simulink model "model"  (R2025b)
settings: Solver=ode4  StartTime=0.0  StopTime=20  FixedStep=1e-3  RelTol=1e-3
values from neighbouring files (symbols this model uses):
  center_circ = [0,0]    [trajectories.m]
  ellipse_center = [0, 0]    [trajectories.m]
  ellipse_x_axis = 3    [trajectories.m]
  ellipse_y_axis = 1    [trajectories.m]
  K_posture = [100;100;0.01]    [posture_controllers.m]    (also in sim_FT.m = [10,10,100]; simulate_full_task.m = [10,10,100])
  KL_params = [1, 1]    [simulate_configuration_control.m]    (also in simulate_trajectory_tracking.m; tracking_controllers.m = [KL_a, KL_xi])
  KNL_b = 100    [sim_FT.m]    (also in simulate_configuration_control.m = 1; simulate_full_task.m; simulate_trajectory_tracking.m = 1; tracking_controllers.m = 1000)
  KNL_xi = 0.25    [sim_FT.m]    (also in simulate_configuration_control.m = 0.5; simulate_full_task.m; simulate_trajectory_tracking.m = 0.5; tracking_controllers.m = 0.9999)
  omega_circ = 1    [trajectories.m]
  q0_posture = [err_mag;err_phase;delta_pos]    [posture_controllers.m]    (also in sim_FT.m = [rho_0; gamma_0; delta_0]; simulate_configuration_control.m; simulate_full_task.m = [rho_0; gamma_0; delta_0])
  q_h_0 = [x_h_0, y_h, theta_h]    [trajectories.m]
  q_h_f = [x_h_f, y_h, theta_h]    [trajectories.m]
  q_v_0 = [x_v, y_v_0, theta_v]    [trajectories.m]
  q_v_f = [x_v, y_v_f, theta_v]    [trajectories.m]
  R_circ = 1    [trajectories.m]
  x0_cartesian = [-1;-1;pi/4]    [posture_controllers.m]    (also in simulate_configuration_control.m)
  zigzag_ampl = 3    [trajectories.m]
  zigzag_period = 6    [trajectories.m]
  zigzag_period_length = 3    [trajectories.m]
settings Model: Creator=llp  LastModifiedBy=fede

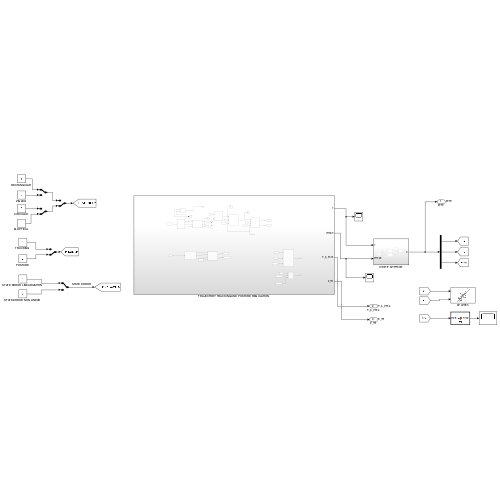
[thumbnail: Simulink's stored preview of the top-level diagram]
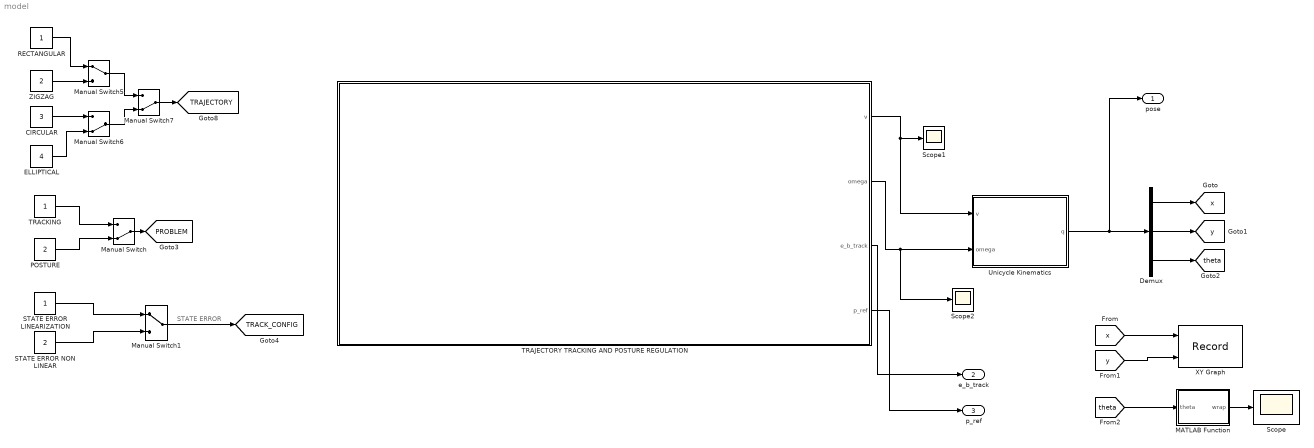
== system model ==
  note: STATE ERROR
  CIRCULAR : Constant  Value=3
  Demux : Demux  Outputs=3
  ELLIPTICAL : Constant  Value=4
  MATLAB Function : MATLAB Function  TreatAsAtomicUnit=on
  Manual Switch : ManualSwitch  CurrentSetting=0
  Manual Switch1 : ManualSwitch
  Manual Switch5 : ManualSwitch
  Manual Switch6 : ManualSwitch  CurrentSetting=0
  Manual Switch7 : ManualSwitch  CurrentSetting=0
  POSTURE : Constant  Value=2
  RECTANGULAR : Constant
  STATE ERROR LINEARIZATION : Constant
  STATE ERROR NON LINEAR : Constant  Value=2
  Scope : Scope
      settings: ActiveDisplayYMinimum=-3.9268154980569436  ActiveDisplayYMaximum=3.926524990405821
  Scope1 : Scope
      settings: ActiveDisplayYMinimum=-1  ActiveDisplayYMaximum=1  DataLoggingVariableName=ScopeData6
  Scope2 : Scope
      settings: ActiveDisplayYMinimum=-1  ActiveDisplayYMaximum=1  DataLoggingVariableName=ScopeData7
  TRACKING : Constant
  TRAJECTORY TRACKING AND POSTURE REGULATION : Subsystem
  Unicycle Kinematics : Subsystem
  XY Graph : Record  NumPorts=2.0  FileSettingsInternal="{\"entries\":[{\"content\":{\"excelSettings\":{\"content\":{},\"type\":\"Streamout.ExcelSettings\"},\"parquetSettings\":{\"content\":{},\"type\":\"Streamout.ParquetSettings\"}},\"type\":\"Streamout.FileSettingStorage\",\"uuid\":\"\"}],\"packageUris\":[\"http:\\/\\/schema.mathworks.com\\/mf0\\/streamout_blocks\\/R2020a\"],\"version\":\"1.0\"}"  FrameSettings=[0, 0]  Layout=[1 1]  SignalsInternal="{\"entries\":[{\"content\":{\"signals\":[{\"content\":{\"blockPath\":[],\"dimensions\":[1,1],\"domain\":\"\",\"lineColor\":\"#a2142f\",\"plots\":[ 1 ],\"port\":1,\"signalID\":1,\"signalName\":\"From\"},\"type\":\"RecordBlkView.Signal\",\"uuid\":\"\"},{\"content\":{\"blockPath\":[],\"dimensions\":[1,1],\"domain\":\"\",\"lineColor\":\"#139fff\",\"plots\":[ 1 ],\"port\":2,\"signalID\":2,\"signalName\":\"From1\"},\"type\":\"RecordBlkView.Signal\",\"uuid\":\"\"}]},\"type\":\"RecordBlkView.InputSignals\",\"uuid\":\"\"}],\"packageUris\":[\"http:\\/\\/schema.mathworks.com\\/mf0\\/streamout_blocks\\/R2020a\"],\"version\":\"1.0\"}"  VisualizationBindings="{\"xyplotplugin\":{\"info\":[{\"series\":[{\"bindingParametersList\":[{\"parameter\":\"X-Axis\",\"signalID\":1,\"signalName\":\"From\"},{\"parameter\":\"Y-Axis\",\"signalID\":2,\"signalName\":\"From1\"}],\"seriesID\":0}],\"subplotID\":1}]}}"  CompatibilityTag=XY
  ZIGZAG : Constant  Value=2
  pose : Outport  SignalName=pose
  e_b_track : Outport  Port=2  SignalName=e_b_track
  p_ref : Outport  Port=3  SignalName=p_ref  PortDimensions=3
  tag scope: PROBLEM=global, TRACK_CONFIG=global, TRAJECTORY=global, theta=global, x=global, y=global
  wires:
  TRACKING/1 -> Manual Switch/1
  POSTURE/1 -> Manual Switch/2
  STATE ERROR LINEARIZATION/1 -> Manual Switch1/1
  STATE ERROR NON LINEAR/1 -> Manual Switch1/2
  Demux/1 -> [x]
  Demux/2 -> [y]
  Demux/3 -> [theta]
  Manual Switch/1 -> [PROBLEM]
  Manual Switch1/1 -> [TRACK_CONFIG]
  [x] -> XY Graph/1
  [y] -> XY Graph/2
  MATLAB Function/1(wrap) -> Scope/1
  [theta] -> MATLAB Function/1(theta)
  RECTANGULAR/1 -> Manual Switch5/1
  ZIGZAG/1 -> Manual Switch5/2
  CIRCULAR/1 -> Manual Switch6/1
  ELLIPTICAL/1 -> Manual Switch6/2
  Manual Switch5/1 -> Manual Switch7/1
  Manual Switch6/1 -> Manual Switch7/2
  Manual Switch7/1 -> [TRAJECTORY]
  TRAJECTORY TRACKING AND POSTURE REGULATION/1(v) -> Unicycle Kinematics/1(v), Scope1/1
  TRAJECTORY TRACKING AND POSTURE REGULATION/2(omega) -> Scope2/1, Unicycle Kinematics/2(omega)
  Unicycle Kinematics/1(q) -> pose/1, Demux/1
  TRAJECTORY TRACKING AND POSTURE REGULATION/3(e_b_track) -> e_b_track/1
  TRAJECTORY TRACKING AND POSTURE REGULATION/4(p_ref) -> p_ref/1

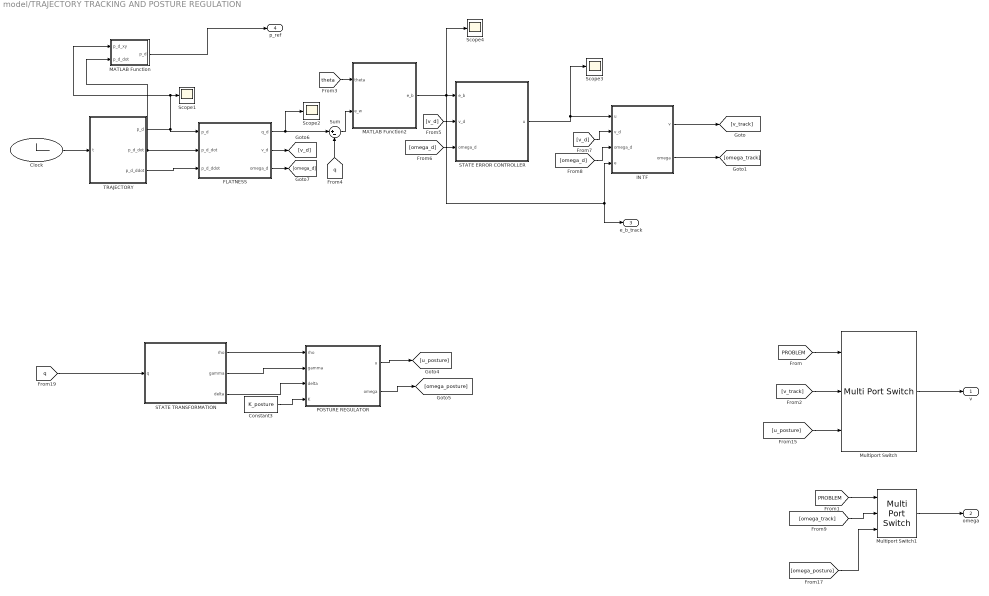
== system model/TRAJECTORY TRACKING AND POSTURE REGULATION ==
  Clock : Clock
  Constant3 : Constant  Value=K_posture
  FLATNESS : MATLAB Function  TreatAsAtomicUnit=on
  IN TF : MATLAB Function  TreatAsAtomicUnit=on
  MATLAB Function : MATLAB Function  TreatAsAtomicUnit=on
  MATLAB Function2 : MATLAB Function  TreatAsAtomicUnit=on
  Multiport Switch : MultiPortSwitch  Inputs=2  SaturateOnIntegerOverflow=off  InputSameDT=off
  Multiport Switch1 : MultiPortSwitch  Inputs=2  SaturateOnIntegerOverflow=off  InputSameDT=off
  POSTURE REGULATOR : MATLAB Function  TreatAsAtomicUnit=on
  STATE ERROR CONTROLLER : Subsystem
  STATE TRANSFORMATION : MATLAB Function  TreatAsAtomicUnit=on
  Scope{1..4} (4 alike) : Scope
      Scope1 settings: ActiveDisplayYMinimum=-1  ActiveDisplayYMaximum=1
      Scope2 settings: ActiveDisplayYMinimum=-1  ActiveDisplayYMaximum=1  DataLoggingVariableName=ScopeData2
      Scope3 settings: ActiveDisplayYMinimum=-1  ActiveDisplayYMaximum=1  DataLoggingVariableName=ScopeData3
      Scope4 settings: ActiveDisplayYMinimum=-4.638821975568507  ActiveDisplayYMaximum=5.2011167151514961  DataLoggingVariableName=ScopeData4
  Sum : Sum  Inputs=|+-
  TRAJECTORY : Subsystem
  v : Outport
  omega : Outport  Port=2
  e_b_track : Outport  Port=3
  p_ref : Outport  Port=4
  wires:
  [v_d] -> STATE ERROR CONTROLLER/2(v_d)
  [omega_d] -> IN TF/3(omega_d)
  STATE ERROR CONTROLLER/1(u) -> Scope3/1, IN TF/1(u)
  [theta] -> MATLAB Function2/1(theta)
  [q] -> Sum/2
  FLATNESS/1(q_d) -> Scope2/1, Sum/1
  Clock/1 -> TRAJECTORY/1(t)
  TRAJECTORY/2(p_d_dot) -> MATLAB Function/2(p_d_dot), FLATNESS/2(p_d_dot)
  FLATNESS/3(omega_d) -> [omega_d]
  MATLAB Function2/1(e_b) -> STATE ERROR CONTROLLER/1(e_b), e_b_track/1, IN TF/4(e), Scope4/1
  TRAJECTORY/3(p_d_ddot) -> FLATNESS/3(p_d_ddot)
  FLATNESS/2(v_d) -> [v_d]
  TRAJECTORY/1(p_d) -> MATLAB Function/1(p_d_xy), Scope1/1, FLATNESS/1(p_d)
  [v_d] -> IN TF/2(v_d)
  [omega_d] -> STATE ERROR CONTROLLER/3(omega_d)
  Sum/1 -> MATLAB Function2/2(e_w)
  Multiport Switch/1 -> v/1
  Multiport Switch1/1 -> omega/1
  [PROBLEM] -> Multiport Switch/1
  [PROBLEM] -> Multiport Switch1/1
  IN TF/1(v) -> [v_track]
  IN TF/2(omega) -> [omega_track]
  [v_track] -> Multiport Switch/2
  [omega_track] -> Multiport Switch1/2
  [u_posture] -> Multiport Switch/3
  [omega_posture] -> Multiport Switch1/3
  POSTURE REGULATOR/1(u) -> [u_posture]
  POSTURE REGULATOR/2(omega) -> [omega_posture]
  [q] -> STATE TRANSFORMATION/1(q)
  STATE TRANSFORMATION/1(rho) -> POSTURE REGULATOR/1(rho)
  STATE TRANSFORMATION/2(gamma) -> POSTURE REGULATOR/2(gamma)
  STATE TRANSFORMATION/3(delta) -> POSTURE REGULATOR/3(delta)
  Constant3/1 -> POSTURE REGULATOR/4(K)
  MATLAB Function/1(p_d) -> p_ref/1

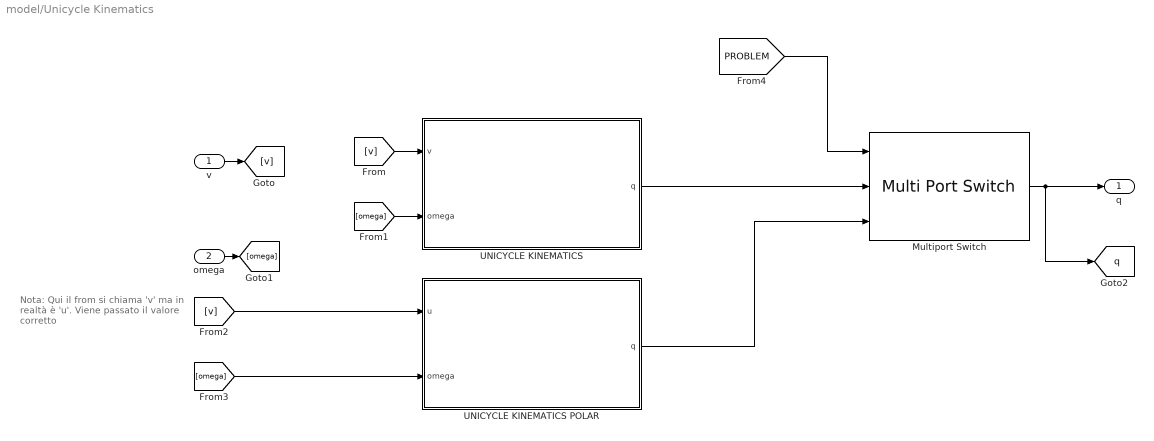
== system model/Unicycle Kinematics ==
  note: Nota: Qui il from si chiama 'v' ma in
      | realtà è 'u'. Viene passato il valore
      | corretto
  v : Inport
  omega : Inport  Port=2
  Multiport Switch : MultiPortSwitch  Inputs=2  SaturateOnIntegerOverflow=off  InputSameDT=off
  UNICYCLE KINEMATICS : Subsystem
  UNICYCLE KINEMATICS POLAR : Subsystem
  q : Outport
  tag scope: q=global
  wires:
  Multiport Switch/1 -> [q], q/1
  UNICYCLE KINEMATICS/1(q) -> Multiport Switch/2
  v/1 -> [v]
  omega/1 -> [omega]
  [omega] -> UNICYCLE KINEMATICS/2(omega)
  [v] -> UNICYCLE KINEMATICS/1(v)
  [v] -> UNICYCLE KINEMATICS POLAR/1(u)
  [omega] -> UNICYCLE KINEMATICS POLAR/2(omega)
  [PROBLEM] -> Multiport Switch/1
  UNICYCLE KINEMATICS POLAR/1(q) -> Multiport Switch/3

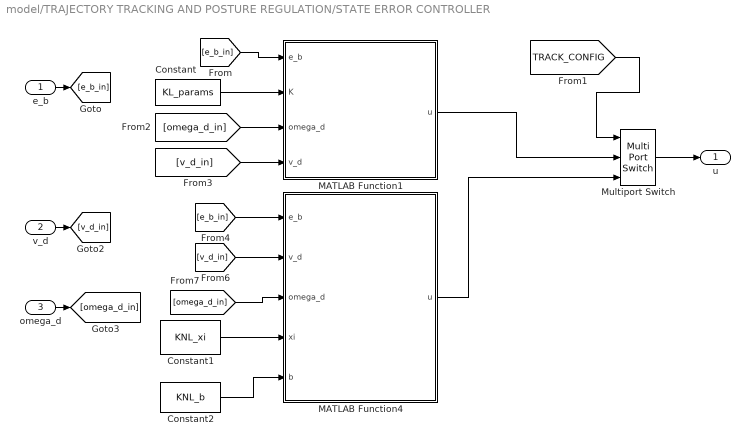
== system model/TRAJECTORY TRACKING AND POSTURE REGULATION/STATE ERROR CONTROLLER ==
  e_b : Inport
  v_d : Inport  Port=2
  omega_d : Inport  Port=3
  Constant : Constant  Value=KL_params
  Constant1 : Constant  Value=KNL_xi
  Constant2 : Constant  Value=KNL_b
  MATLAB Function1 : MATLAB Function  TreatAsAtomicUnit=on
  MATLAB Function4 : MATLAB Function  TreatAsAtomicUnit=on
  Multiport Switch : MultiPortSwitch  Inputs=2  SaturateOnIntegerOverflow=off  InputSameDT=off
  u : Outport
  wires:
  [v_d_in] -> MATLAB Function4/2(v_d)
  [omega_d_in] -> MATLAB Function4/3(omega_d)
  e_b/1 -> [e_b_in]
  v_d/1 -> [v_d_in]
  omega_d/1 -> [omega_d_in]
  [e_b_in] -> MATLAB Function1/1(e_b)
  [e_b_in] -> MATLAB Function4/1(e_b)
  Multiport Switch/1 -> u/1
  Constant/1 -> MATLAB Function1/2(K)
  Constant1/1 -> MATLAB Function4/4(xi)
  Constant2/1 -> MATLAB Function4/5(b)
  MATLAB Function1/1(u) -> Multiport Switch/2
  MATLAB Function4/1(u) -> Multiport Switch/3
  [TRACK_CONFIG] -> Multiport Switch/1
  [omega_d_in] -> MATLAB Function1/3(omega_d)
  [v_d_in] -> MATLAB Function1/4(v_d)

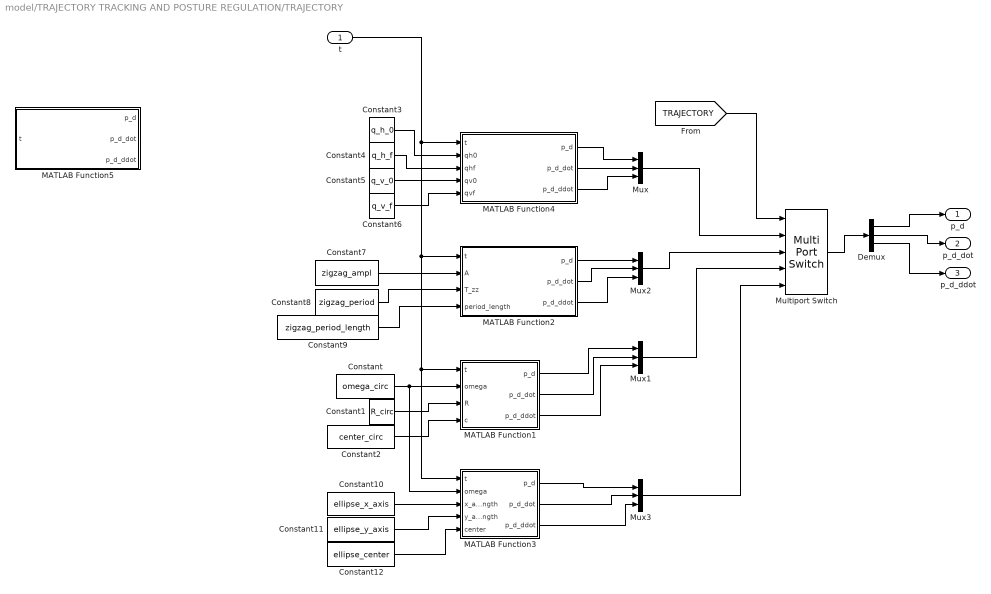
== system model/TRAJECTORY TRACKING AND POSTURE REGULATION/TRAJECTORY ==
  t : Inport
  Constant : Constant  Value=omega_circ
  Constant1 : Constant  Value=R_circ
  Constant10 : Constant  Value=ellipse_x_axis
  Constant11 : Constant  Value=ellipse_y_axis
  Constant12 : Constant  Value=ellipse_center
  Constant2 : Constant  Value=center_circ
  Constant3 : Constant  Value=q_h_0
  Constant4 : Constant  Value=q_h_f
  Constant5 : Constant  Value=q_v_0
  Constant6 : Constant  Value=q_v_f
  Constant7 : Constant  Value=zigzag_ampl
  Constant8 : Constant  Value=zigzag_period
  Constant9 : Constant  Value=zigzag_period_length
  Demux : Demux  Outputs=3
  MATLAB Function1 : MATLAB Function  TreatAsAtomicUnit=on
  MATLAB Function2 : MATLAB Function  TreatAsAtomicUnit=on
  MATLAB Function3 : MATLAB Function  TreatAsAtomicUnit=on
  MATLAB Function4 : MATLAB Function  TreatAsAtomicUnit=on
  MATLAB Function5 : MATLAB Function  TreatAsAtomicUnit=on
  Multiport Switch : MultiPortSwitch  Inputs=4  SaturateOnIntegerOverflow=off  InputSameDT=off
  Mux{,1..3} (4 alike) : Mux  Inputs=3
  p_d : Outport
  p_d_dot : Outport  Port=2
  p_d_ddot : Outport  Port=3
  wires:
  Constant6/1 -> MATLAB Function4/5(qvf)
  t/1 -> MATLAB Function4/1(t), MATLAB Function1/1(t), MATLAB Function3/1(t), MATLAB Function2/1(t)
  Constant2/1 -> MATLAB Function1/4(c)
  Constant3/1 -> MATLAB Function4/2(qh0)
  Constant/1 -> MATLAB Function1/2(omega), MATLAB Function3/2(omega)
  Constant5/1 -> MATLAB Function4/4(qv0)
  Constant4/1 -> MATLAB Function4/3(qhf)
  Constant1/1 -> MATLAB Function1/3(R)
  MATLAB Function4/1(p_d) -> Mux/1
  MATLAB Function4/2(p_d_dot) -> Mux/2
  MATLAB Function4/3(p_d_ddot) -> Mux/3
  Mux/1 -> Multiport Switch/2
  [TRAJECTORY] -> Multiport Switch/1
  Multiport Switch/1 -> Demux/1
  Demux/1 -> p_d/1
  Demux/2 -> p_d_dot/1
  Demux/3 -> p_d_ddot/1
  MATLAB Function1/1(p_d) -> Mux1/1
  MATLAB Function1/2(p_d_dot) -> Mux1/2
  MATLAB Function1/3(p_d_ddot) -> Mux1/3
  MATLAB Function2/1(p_d) -> Mux2/1
  MATLAB Function2/3(p_d_ddot) -> Mux2/3
  MATLAB Function2/2(p_d_dot) -> Mux2/2
  Mux1/1 -> Multiport Switch/4
  MATLAB Function3/1(p_d) -> Mux3/1
  MATLAB Function3/2(p_d_dot) -> Mux3/2
  MATLAB Function3/3(p_d_ddot) -> Mux3/3
  Mux3/1 -> Multiport Switch/5
  Mux2/1 -> Multiport Switch/3
  Constant9/1 -> MATLAB Function2/4(period_length)
  Constant8/1 -> MATLAB Function2/3(T_zz)
  Constant7/1 -> MATLAB Function2/2(A)
  Constant10/1 -> MATLAB Function3/3(x_axis_length)
  Constant11/1 -> MATLAB Function3/4(y_axis_length)
  Constant12/1 -> MATLAB Function3/5(center)

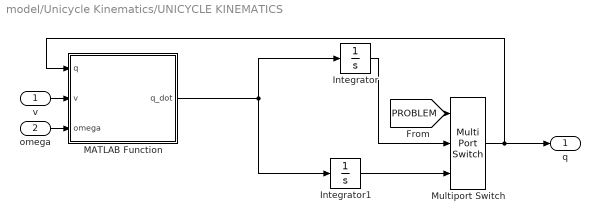
== system model/Unicycle Kinematics/UNICYCLE KINEMATICS ==
  v : Inport
  omega : Inport  Port=2
  Integrator : Integrator
  Integrator1 : Integrator  InitialCondition=x0_cartesian
  MATLAB Function : MATLAB Function  TreatAsAtomicUnit=on
  Multiport Switch : MultiPortSwitch  Inputs=2  SaturateOnIntegerOverflow=off  InputSameDT=off
  q : Outport
  wires:
  v/1 -> MATLAB Function/2(v)
  omega/1 -> MATLAB Function/3(omega)
  MATLAB Function/1(q_dot) -> Integrator1/1, Integrator/1
  [PROBLEM] -> Multiport Switch/1
  Integrator1/1 -> Multiport Switch/3
  Integrator/1 -> Multiport Switch/2
  Multiport Switch/1 -> MATLAB Function/1(q), q/1

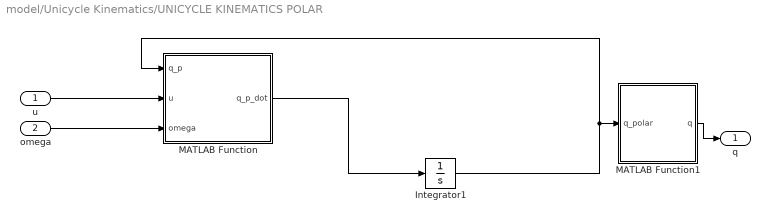
== system model/Unicycle Kinematics/UNICYCLE KINEMATICS POLAR ==
  u : Inport
  omega : Inport  Port=2
  Integrator1 : Integrator  InitialCondition=q0_posture
  MATLAB Function : MATLAB Function  TreatAsAtomicUnit=on
  MATLAB Function1 : MATLAB Function  TreatAsAtomicUnit=on
  q : Outport
  wires:
  u/1 -> MATLAB Function/2(u)
  omega/1 -> MATLAB Function/3(omega)
  MATLAB Function/1(q_p_dot) -> Integrator1/1
  Integrator1/1 -> MATLAB Function1/1(q_polar), MATLAB Function/1(q_p)
  MATLAB Function1/1(q) -> q/1

== matlab function model/TRAJECTORY TRACKING AND POSTURE REGULATION/TRAJECTORY/MATLAB Function4 ==
  data: t input; p_d output; p_d_dot output; p_d_ddot output; qh0 input; qhf input; qv0 input; qvf input
function [p_d, p_d_dot, p_d_ddot] = rectangular_traj(t, qh0, qhf, qv0, qvf)
    % Extract values from your defined vectors
    x_start = qh0(1);
    y_start = qh0(2);
    x_end   = qhf(1);
    y_end   = qvf(2); % Height from the vertical segment definition
    
    L_h = x_end - x_start;
    L_v = y_end - y_start;
    
    T_side = 20 / 4; % 2.5 seconds per side
    v_h = L_h / T_side;
    v_v = L_v / T_side;

    if t < T_side
        % Side 1: Bottom (Right)
        x = x_start + v_h * t;
        y = y_start;
        vx = v_h; vy = 0;
    elseif t < 2*T_side
        % Side 2: Right (Up)
        x = x_end;
        y = y_start + v_v * (t - T_side);
        vx = 0; vy = v_v;
    elseif t < 3*T_side
        % Side 3: Top (Left)
        x = x_end - v_h * (t - 2*T_side);
        y = y_end;
        vx = -v_h; vy = 0;
    else
        % Side 4: Left (Down)
        x = x_start;
        y = y_end - v_v * (t - 3*T_side);
        vx = 0; vy = -v_v;
    end

    p_d = [x; y];
    p_d_dot = [vx; vy];
    p_d_ddot = [0; 0];

end

== matlab function model/TRAJECTORY TRACKING AND POSTURE REGULATION/TRAJECTORY/MATLAB Function2 ==
  data: t input; p_d output; p_d_dot output; p_d_ddot output; A input; T_zz input; period_length input
function [p_d, p_d_dot, p_d_ddot] = zigzag_traj(t, A, T_zz, period_length)
    % A: Amplitude (half-height of the zigzag)
    % T_zz: Period of a full cycle (up and down)
    % period_length: length of a full cycle
    
    t_rel = mod(t, T_zz);
    vy_speed = (4 * A) / T_zz; % Speed required to cover 4*A in T_zz seconds
    
    
    vx = (period_length) / 10;
    x = vx * t;
    
    % Triangle wave logic for Y
    if t_rel < T_zz/4
        % Climbing from 0 to A
        y = vy_speed * t_rel;
        vy = vy_speed;
    elseif t_rel < 3*T_zz/4
        % Falling from A to -A
        y = A - vy_speed * (t_rel - T_zz/4);
        vy = -vy_speed;
    else
        % Climbing from -A back to 0
        y = -A + vy_speed * (t_rel - 3*T_zz/4);
        vy = vy_speed;
    end
    
    p_d = [x; y];
    p_d_dot = [vx; vy];
    p_d_ddot = [0; 0];
end

== matlab function model/TRAJECTORY TRACKING AND POSTURE REGULATION/TRAJECTORY/MATLAB Function3 ==
  data: t input; p_d output; p_d_dot output; p_d_ddot output; omega input; x_axis_length input; y_axis_length input; center input
function [p_d, p_d_dot, p_d_ddot] = elliptical_traj(t, omega, x_axis_length, y_axis_length, center)
    % t: Current time
    % omega: Angular velocity (rad/s)
    % a: Semi-axis length in X
    % b: Semi-axis length in Y
    % c: Center coordinates [xc; yc]

    xc = center(1);
    yc = center(2);

    % Current angle based on time
    theta = omega * t;

    % Position p_d
    x = xc + x_axis_length * cos(theta);
    y = yc + y_axis_length * sin(theta);

    % Velocity p_d_dot (First derivative)
    x_dot = -x_axis_length * omega * sin(theta);
    y_dot =  y_axis_length * omega * cos(theta);

    % Acceleration p_d_ddot (Second derivative)
    x_ddot = -x_axis_length * omega^2 * cos(theta);
    y_ddot = -y_axis_length * omega^2 * sin(theta);

    % Outputs
    p_d = [x; y];
    p_d_dot = [x_dot; y_dot];
    p_d_ddot = [x_ddot; y_ddot];
end

== matlab function model/TRAJECTORY TRACKING AND POSTURE REGULATION/MATLAB Function ==
  data: p_d_xy input; p_d output; p_d_dot input
function p_d = fcn(p_d_xy, p_d_dot)
    x = p_d_xy(1);
    y = p_d_xy(2);
    
    vx = p_d_dot(1);
    vy = p_d_dot(2);
    
    % Heading is the angle of the velocity vector
    theta = atan2(vy, vx); 
    
    p_d = [x; y; theta];
end

== matlab function model/Unicycle Kinematics/UNICYCLE KINEMATICS POLAR/MATLAB Function ==
  data: q_p input; q_p_dot output; u input; omega input
function q_p_dot = fcn(q_p, u, omega)
%write the unicycle model
q_p_dot= zeros(3,1);
rho = q_p(1);
gamma = q_p(2);

q_p_dot(1) = -u*cos(gamma);
q_p_dot(2) = sin(gamma)*u-omega;
q_p_dot(3) = sin(gamma)*u;

== matlab function model/TRAJECTORY TRACKING AND POSTURE REGULATION/POSTURE REGULATOR ==
  data: u output; omega output; rho input; gamma input; delta input; K input
function [u, omega] = posture_regulator(rho, gamma, delta, K)

%u = K(1)*rho*cos(gamma);
u = K(1)*cos(gamma);
omega = K(2)*gamma + K(1)*((sin(gamma)*cos(gamma))/gamma) *(gamma+K(3)*delta);

== matlab function model/TRAJECTORY TRACKING AND POSTURE REGULATION/STATE TRANSFORMATION ==
  data: rho output; q input; gamma output; delta output
function [rho, gamma, delta] = state_tf(q)


x = q(1);
y = q(2);
theta = q(3);

rho = sqrt(x^2+y^2);
gamma = atan2(y,x)+pi-theta;
delta = gamma+theta;

== matlab function model/Unicycle Kinematics/UNICYCLE KINEMATICS POLAR/MATLAB Function1 ==
  data: q_polar input; q output
function q = inv_state_tf(q_polar)

rho = q_polar(1);
gamma = q_polar(2);
delta = q_polar(3);


x = -rho*cos(delta);
y = -rho*sin(delta);
theta = delta - gamma;

q = [x; y; theta];

== matlab function model/TRAJECTORY TRACKING AND POSTURE REGULATION/STATE ERROR CONTROLLER/MATLAB Function1 ==
  data: e_b input; u output; K input size=[1 2]; omega_d input; v_d input
function u = linear_gain(e_b, K, omega_d, v_d)

a = K(1);
xi = K(2);

K1 = 2*xi*a;
K3 = 2*xi*a;
K2 = (a^2-omega_d^2)/(v_d);


u = zeros(2,1);
u(1) = -K1*e_b(1);
u(2) = -K2*e_b(2)-K3*e_b(3);

== matlab function model/Unicycle Kinematics/UNICYCLE KINEMATICS/MATLAB Function ==
  data: q input; q_dot output; v input; omega input
function q_dot = fcn(q, v, omega)
%write the unicycle model
q_dot= zeros(3,1);

q_dot(1) = v*cos(q(3));
q_dot(2) = v*sin(q(3));
q_dot(3) = omega;

== matlab function model/MATLAB Function ==
  data: theta input; wrap output
function wrap = fcn(theta)

wrap = mod(theta+pi,2*pi)-pi ;

== matlab function model/TRAJECTORY TRACKING AND POSTURE REGULATION/MATLAB Function2 ==
  data: theta input; e_b output; e_w input
function e_b = Rz(theta, e_w)

e_b = zeros(3,1);
e_b(1)=cos(theta)*e_w(1)+sin(theta)*e_w(2);
e_b(2)=-sin(theta)*e_w(1)+cos(theta)*e_w(2);
e_b(3)=e_w(3);

== matlab function model/TRAJECTORY TRACKING AND POSTURE REGULATION/IN TF ==
  data: u input; v output; omega output; v_d input; omega_d input; e input
function [v, omega] = input_transformation(u, v_d, omega_d,e)
%initialization
v= 0;
omega = 0;
%calcolo di v e omega, come mostrato in slide 19
v = v_d*cos(e(3))-u(1);
omega = omega_d-u(2);

== matlab function model/TRAJECTORY TRACKING AND POSTURE REGULATION/STATE ERROR CONTROLLER/MATLAB Function4 ==
  data: e_b input; u output; v_d input; omega_d input size=1; xi input size=1; b input size=1
function u = nonlinear_gain(e_b, v_d, omega_d, xi, b)

K2 = b;
K1 = 2*xi*sqrt(b*v_d+omega_d^2);
K3 = 2*xi*sqrt(b*v_d+omega_d^2);

u=zeros(2,1);
u(1) = -K1*e_b(1);
u(2) = -K2*v_d*e_b(2)*sin(e_b(3))/(sign(e_b(3))*sqrt((e_b(3)+1e-6)^2))-K3*e_b(3);

% Angular velocity command (with singularity protection)
% Use a threshold to avoid division by zero
if abs(e_b(3)) < 1e-5
    % Limit: sin(x)/x as x -> 0 is 1
    sinc = 1.0;
else
    sinc = sin(e_b(3)) / e_b(3);
end

% u(2) = -K2 * v_d * e_b(2) * [sin(e_theta)/e_theta] - K3 * e_theta
u(2) = -K2 * v_d * e_b(2) * sinc - K3 * e_b(3);

== matlab function model/TRAJECTORY TRACKING AND POSTURE REGULATION/FLATNESS ==
  data: p_d input; q_d output; v_d output; omega_d output; p_d_dot input; p_d_ddot input
function [q_d, v_d, omega_d] = flatness(p_d, p_d_dot, p_d_ddot)

x = p_d(1);
y = p_d(2);

x_dot = p_d_dot(1);
y_dot = p_d_dot(2);

x_ddot = p_d_ddot(1);
y_ddot = p_d_ddot(2);

% velocità
v_d = sqrt(x_dot^2 + y_dot^2);

% orientamento
theta_d = atan2(y_dot, x_dot);

% velocità angolare
den = x_dot^2 + y_dot^2;

if den < 1e-8
    omega_d = 0;
else
    omega_d = (x_dot*y_ddot - y_dot*x_ddot)/den;
end

% stato desiderato
q_d = [x; y; theta_d];

end

== matlab function model/TRAJECTORY TRACKING AND POSTURE REGULATION/TRAJECTORY/MATLAB Function1 ==
  data: t input; p_d output; p_d_dot output; p_d_ddot output; omega input; R input; c input
function [p_d, p_d_dot, p_d_ddot] = circular_traj(t,omega,R,c)

xc = c(1);
yc = c(2);


theta = omega*t;

x = xc + R*cos(theta);
y = yc + R*sin(theta);

x_dot = -R*omega*sin(theta);
y_dot =  R*omega*cos(theta);

x_ddot = -R*omega^2*cos(theta);
y_ddot = -R*omega^2*sin(theta);

p_d = [x; y];
p_d_dot = [x_dot; y_dot];
p_d_ddot = [x_ddot; y_ddot];

end

== matlab function model/TRAJECTORY TRACKING AND POSTURE REGULATION/TRAJECTORY/MATLAB Function5 ==
  data: t input; p_d output; p_d_dot output; p_d_ddot output
function [p_d, p_d_dot, p_d_ddot] = horizontal_traj(t)

x0 = 0;
y0 = 0;

v = 1;  
x = x0 + v*t;
y = y0;

x_dot = v;
y_dot = 0;

x_ddot = 0;
y_ddot = 0;

p_d = [x; y];
p_d_dot = [x_dot; y_dot];
p_d_ddot = [x_ddot; y_ddot];

end
